simulink model "db3_7_Level_double"  (R2021a)
settings: Solver=VariableStepAuto  StartTime=0.0  StopTime=8  RelTol=1e-3
undefined symbols (not defined in the file): lambda2
libraries: dspsigops x15, dspquant2 x1
(part 2 of 4)

== system db3_7_Level_double/1st_Level_Decomp/HiD_Odd ==
  In_HiD_o : Inport  OutDataTypeStr=double  SampleTime=1/44100
  Add : Sum  AccumDataTypeStr=double  OutDataTypeStr=double
  Add1 : Sum  AccumDataTypeStr=double  OutDataTypeStr=double
  Delay{,1..3} (4 alike) : Delay  DelayLength=1  SampleTime=1/44100
  HiD_1 : Constant  Value=0.806891509  OutDataTypeStr=double  SampleTime=1/44100
  HiD_3 : Constant  Value=-0.13501102  OutDataTypeStr=double  SampleTime=1/44100
  HiD_5 : Constant  Value=0.035226292  OutDataTypeStr=double  SampleTime=1/44100
  Multiply : Product  OutDataTypeStr=double
  Multiply1 : Product  OutDataTypeStr=double
  Multiply2 : Product  OutDataTypeStr=double
  Rate Transition : RateTransition  OutPortSampleTime=1/44100
  Rate Transition1 : RateTransition  OutPortSampleTime=1/44100
  Out_HiD_o : Outport  OutDataTypeStr=double  SampleTime=1/44100  VectorParamsAs1DForOutWhenUnconnected=off
  wires:
  HiD_5/1 -> Multiply2/1
  HiD_3/1 -> Multiply1/1
  Add/1 -> Out_HiD_o/1
  Delay2/1 -> Add1/2
  Delay3/1 -> Add/2
  Add1/1 -> Delay3/1
  Multiply/1 -> Add/1
  HiD_1/1 -> Multiply/1
  Rate Transition/1 -> Delay1/1, Multiply1/2
  Multiply1/1 -> Add1/1
  Multiply2/1 -> Delay2/1
  Rate Transition1/1 -> Multiply2/2
  In_HiD_o/1 -> Multiply/2, Delay/1
  Delay/1 -> Rate Transition/1
  Delay1/1 -> Rate Transition1/1

== system db3_7_Level_double/1st_Level_Decomp/LoD_Even ==
  In_LoD_e : Inport  OutDataTypeStr=double  SampleTime=1/44100
  Add : Sum  AccumDataTypeStr=double  OutDataTypeStr=double
  Add1 : Sum  AccumDataTypeStr=double  OutDataTypeStr=double
  Delay{,1..3} (4 alike) : Delay  DelayLength=1  SampleTime=1/44100
  LoD_0 : Constant  Value=0.035226292  OutDataTypeStr=double  SampleTime=1/44100
  LoD_2 : Constant  Value=-0.13501102  OutDataTypeStr=double  SampleTime=1/44100
  LoD_4 : Constant  Value=0.806891509  OutDataTypeStr=double  SampleTime=1/44100
  Multiply : Product  OutDataTypeStr=double
  Multiply1 : Product  OutDataTypeStr=double
  Multiply2 : Product  OutDataTypeStr=double
  Rate Transition : RateTransition  OutPortSampleTime=1/44100
  Rate Transition1 : RateTransition  OutPortSampleTime=1/44100
  Out_LoD_e : Outport  OutDataTypeStr=double  SampleTime=1/44100  VectorParamsAs1DForOutWhenUnconnected=off
  wires:
  LoD_4/1 -> Multiply2/1
  LoD_2/1 -> Multiply1/1
  Add/1 -> Out_LoD_e/1
  Delay2/1 -> Add1/2
  Delay3/1 -> Add/2
  Add1/1 -> Delay3/1
  Multiply/1 -> Add/1
  LoD_0/1 -> Multiply/1
  Rate Transition/1 -> Delay1/1, Multiply1/2
  Multiply1/1 -> Add1/1
  Multiply2/1 -> Delay2/1
  Rate Transition1/1 -> Multiply2/2
  In_LoD_e/1 -> Delay/1, Multiply/2
  Delay/1 -> Rate Transition/1
  Delay1/1 -> Rate Transition1/1

== system db3_7_Level_double/1st_Level_Decomp/LoD_Odd ==
  In_LoD_o : Inport  OutDataTypeStr=double  SampleTime=1/44100
  Add : Sum  AccumDataTypeStr=double  OutDataTypeStr=double
  Add1 : Sum  AccumDataTypeStr=double  OutDataTypeStr=double
  Delay{,1..3} (4 alike) : Delay  DelayLength=1  SampleTime=1/44100
  LoD_1 : Constant  Value=-0.085441274  OutDataTypeStr=double  SampleTime=1/44100
  LoD_3 : Constant  Value=0.459877502  OutDataTypeStr=double  SampleTime=1/44100
  LoD_5 : Constant  Value=0.332670553  OutDataTypeStr=double  SampleTime=1/44100
  Multiply : Product  OutDataTypeStr=double
  Multiply1 : Product  OutDataTypeStr=double
  Multiply2 : Product  OutDataTypeStr=double
  Rate Transition : RateTransition  OutPortSampleTime=1/44100
  Rate Transition1 : RateTransition  OutPortSampleTime=1/44100
  Out_LoD_o : Outport  OutDataTypeStr=double  SampleTime=1/44100  VectorParamsAs1DForOutWhenUnconnected=off
  wires:
  LoD_5/1 -> Multiply2/1
  LoD_3/1 -> Multiply1/1
  Add/1 -> Out_LoD_o/1
  Delay2/1 -> Add1/2
  Delay3/1 -> Add/2
  Add1/1 -> Delay3/1
  Multiply/1 -> Add/1
  LoD_1/1 -> Multiply/1
  Rate Transition/1 -> Delay1/1, Multiply1/2
  Multiply1/1 -> Add1/1
  Multiply2/1 -> Delay2/1
  Rate Transition1/1 -> Multiply2/2
  In_LoD_o/1 -> Delay/1, Multiply/2
  Delay/1 -> Rate Transition/1
  Delay1/1 -> Rate Transition1/1

== system db3_7_Level_double/1st_Level_Recon/HiR_Even ==
  In_HiR_e : Inport  OutDataTypeStr=double  SampleTime=1/44100
  Add : Sum  AccumDataTypeStr=double  OutDataTypeStr=double
  Add1 : Sum  AccumDataTypeStr=double  OutDataTypeStr=double
  Delay : Delay  DelayLength=1  SampleTime=1/44100
  Delay1 : Delay  DelayLength=1  SampleTime=1/44100
  Delay2 : Delay  DelayLength=1  SampleTime=0.000022675736
  Delay3 : Delay  DelayLength=1  SampleTime=0.000022675736
  HiR_0 : Constant  Value=0.035226292  OutDataTypeStr=double  SampleTime=1/44100
  HiR_2 : Constant  Value=-0.13501102  OutDataTypeStr=double  SampleTime=1/44100
  HiR_4 : Constant  Value=0.806891509  OutDataTypeStr=double  SampleTime=1/44100
  Multiply : Product  OutDataTypeStr=double
  Multiply1 : Product  OutDataTypeStr=double
  Multiply2 : Product  OutDataTypeStr=double
  Rate Transition : RateTransition  OutPortSampleTime=1/44100
  Rate Transition1 : RateTransition  OutPortSampleTime=1/44100
  Out_HiR_e : Outport  OutDataTypeStr=double  SampleTime=1/44100  VectorParamsAs1DForOutWhenUnconnected=off
  wires:
  Delay3/1 -> Add/2
  In_HiR_e/1 -> Delay/1, Multiply/2
  HiR_4/1 -> Multiply2/1
  Multiply/1 -> Add/1
  Add1/1 -> Delay3/1
  Multiply2/1 -> Delay2/1
  Multiply1/1 -> Add1/1
  Delay2/1 -> Add1/2
  Add/1 -> Out_HiR_e/1
  HiR_0/1 -> Multiply/1
  HiR_2/1 -> Multiply1/1
  Delay1/1 -> Rate Transition1/1
  Rate Transition/1 -> Delay1/1, Multiply1/2
  Rate Transition1/1 -> Multiply2/2
  Delay/1 -> Rate Transition/1

== system db3_7_Level_double/1st_Level_Recon/HiR_Odd ==
  In_HiR_o : Inport  OutDataTypeStr=double  SampleTime=1/44100
  Add : Sum  AccumDataTypeStr=double  OutDataTypeStr=double
  Add1 : Sum  AccumDataTypeStr=double  OutDataTypeStr=double
  Delay{,1..3} (4 alike) : Delay  DelayLength=1  SampleTime=1/44100
  HiR_1 : Constant  Value=0.085441274  OutDataTypeStr=double  SampleTime=1/44100
  HiR_3 : Constant  Value=-0.459877502  OutDataTypeStr=double  SampleTime=1/44100
  HiR_5 : Constant  Value=-0.332670553  OutDataTypeStr=double  SampleTime=1/44100  LockScale=on
  Multiply : Product  OutDataTypeStr=double
  Multiply1 : Product  OutDataTypeStr=double
  Multiply2 : Product  OutDataTypeStr=double
  Rate Transition : RateTransition  OutPortSampleTime=1/44100
  Rate Transition1 : RateTransition  OutPortSampleTime=1/44100
  Out_HiR_o : Outport  OutDataTypeStr=double  SampleTime=1/44100  VectorParamsAs1DForOutWhenUnconnected=off
  wires:
  Delay/1 -> Rate Transition/1
  Rate Transition1/1 -> Multiply2/2
  Delay2/1 -> Add1/2
  HiR_1/1 -> Multiply/1
  Add/1 -> Out_HiR_o/1
  Delay1/1 -> Rate Transition1/1
  HiR_3/1 -> Multiply1/1
  Multiply1/1 -> Add1/1
  Rate Transition/1 -> Delay1/1, Multiply1/2
  Add1/1 -> Delay3/1
  Multiply/1 -> Add/1
  In_HiR_o/1 -> Delay/1, Multiply/2
  Multiply2/1 -> Delay2/1
  HiR_5/1 -> Multiply2/1
  Delay3/1 -> Add/2

== system db3_7_Level_double/1st_Level_Recon/LoR_Even ==
  In_LoR_e : Inport  OutDataTypeStr=double  SampleTime=1/44100
  Add : Sum  AccumDataTypeStr=double  OutDataTypeStr=double
  Add1 : Sum  AccumDataTypeStr=double  OutDataTypeStr=double
  Delay{,1..3} (4 alike) : Delay  DelayLength=1  SampleTime=1/44100
  LoR_0 : Constant  Value=0.332670553  OutDataTypeStr=double  SampleTime=1/44100
  LoR_2 : Constant  Value=0.459877502  OutDataTypeStr=double  SampleTime=1/44100
  LoR_4 : Constant  Value=-0.085441274  OutDataTypeStr=double  SampleTime=1/44100
  Multiply : Product  OutDataTypeStr=double
  Multiply1 : Product  OutDataTypeStr=double
  Multiply2 : Product  OutDataTypeStr=double
  Rate Transition : RateTransition  OutPortSampleTime=1/44100
  Rate Transition1 : RateTransition  OutPortSampleTime=1/44100
  Out_LoR_e : Outport  OutDataTypeStr=double  SampleTime=1/44100  VectorParamsAs1DForOutWhenUnconnected=off
  wires:
  Delay/1 -> Rate Transition/1
  Rate Transition1/1 -> Multiply2/2
  Delay2/1 -> Add1/2
  LoR_0/1 -> Multiply/1
  Add/1 -> Out_LoR_e/1
  Delay1/1 -> Rate Transition1/1
  LoR_2/1 -> Multiply1/1
  Multiply1/1 -> Add1/1
  Rate Transition/1 -> Delay1/1, Multiply1/2
  Add1/1 -> Delay3/1
  Multiply/1 -> Add/1
  In_LoR_e/1 -> Delay/1, Multiply/2
  Multiply2/1 -> Delay2/1
  LoR_4/1 -> Multiply2/1
  Delay3/1 -> Add/2

== system db3_7_Level_double/1st_Level_Recon/LoR_Odd ==
  In_LoR_o : Inport  OutDataTypeStr=double  SampleTime=1/44100
  Add : Sum  AccumDataTypeStr=double  OutDataTypeStr=double
  Add1 : Sum  AccumDataTypeStr=double  OutDataTypeStr=double
  Delay{,1..3} (4 alike) : Delay  DelayLength=1  SampleTime=1/44100
  LoR_1 : Constant  Value=0.806891509  OutDataTypeStr=double  SampleTime=1/44100
  LoR_3 : Constant  Value=-0.13501102  OutDataTypeStr=double  SampleTime=1/44100
  LoR_5 : Constant  Value=0.035226292  OutDataTypeStr=double  SampleTime=1/44100
  Multiply : Product  OutDataTypeStr=double
  Multiply1 : Product  OutDataTypeStr=double
  Multiply2 : Product  OutDataTypeStr=double
  Rate Transition : RateTransition  OutPortSampleTime=1/44100
  Rate Transition1 : RateTransition  OutPortSampleTime=1/44100
  Out_LoR_o : Outport  OutDataTypeStr=double  SampleTime=1/44100  VectorParamsAs1DForOutWhenUnconnected=off
  wires:
  Delay/1 -> Rate Transition/1
  Rate Transition1/1 -> Multiply2/2
  Delay2/1 -> Add1/2
  LoR_1/1 -> Multiply/1
  Add/1 -> Out_LoR_o/1
  Delay1/1 -> Rate Transition1/1
  LoR_3/1 -> Multiply1/1
  Multiply1/1 -> Add1/1
  Rate Transition/1 -> Delay1/1, Multiply1/2
  Add1/1 -> Delay3/1
  Multiply/1 -> Add/1
  In_LoR_o/1 -> Delay/1, Multiply/2
  Multiply2/1 -> Delay2/1
  LoR_5/1 -> Multiply2/1
  Delay3/1 -> Add/2

== system db3_7_Level_double/2nd_Level_Decomp/HiD_Even ==
  In_HiD_e : Inport  OutDataTypeStr=double  SampleTime=1/44100
  Add : Sum  AccumDataTypeStr=double  OutDataTypeStr=double
  Add1 : Sum  AccumDataTypeStr=double  OutDataTypeStr=double
  Delay{,1..3} (4 alike) : Delay  DelayLength=1  SampleTime=1/44100
  HiD_0 : Constant  Value=-0.332670553  OutDataTypeStr=double  SampleTime=1/44100
  HiD_2 : Constant  Value=-0.459877502  OutDataTypeStr=double  SampleTime=1/44100
  HiD_4 : Constant  Value=0.085441274  OutDataTypeStr=double  SampleTime=1/44100
  Multiply : Product  OutDataTypeStr=double
  Multiply1 : Product  OutDataTypeStr=double
  Multiply2 : Product  OutDataTypeStr=double
  Rate Transition : RateTransition  OutPortSampleTime=1/44100
  Rate Transition1 : RateTransition  OutPortSampleTime=1/44100
  Out_HiD_e : Outport  OutDataTypeStr=double  SampleTime=1/44100  VectorParamsAs1DForOutWhenUnconnected=off
  wires:
  In_HiD_e/1 -> Delay/1, Multiply/2
  Rate Transition/1 -> Delay1/1, Multiply1/2
  HiD_0/1 -> Multiply/1
  HiD_2/1 -> Multiply1/1
  Add/1 -> Out_HiD_e/1
  Rate Transition1/1 -> Multiply2/2
  HiD_4/1 -> Multiply2/1
  Multiply1/1 -> Add1/1
  Multiply2/1 -> Delay2/1
  Delay2/1 -> Add1/2
  Add1/1 -> Delay3/1
  Delay3/1 -> Add/2
  Multiply/1 -> Add/1
  Delay/1 -> Rate Transition/1
  Delay1/1 -> Rate Transition1/1

== system db3_7_Level_double/2nd_Level_Decomp/HiD_Odd ==
  In_HiD_o : Inport  OutDataTypeStr=double  SampleTime=1/44100
  Add : Sum  AccumDataTypeStr=double  OutDataTypeStr=double
  Add1 : Sum  AccumDataTypeStr=double  OutDataTypeStr=double
  Delay{,1..3} (4 alike) : Delay  DelayLength=1  SampleTime=1/44100
  HiD_1 : Constant  Value=0.806891509  OutDataTypeStr=double  SampleTime=1/44100
  HiD_3 : Constant  Value=-0.13501102  OutDataTypeStr=double  SampleTime=1/44100
  HiD_5 : Constant  Value=0.035226292  OutDataTypeStr=double  SampleTime=1/44100
  Multiply : Product  OutDataTypeStr=double
  Multiply1 : Product  OutDataTypeStr=double
  Multiply2 : Product  OutDataTypeStr=double
  Rate Transition : RateTransition  OutPortSampleTime=1/44100
  Rate Transition1 : RateTransition  OutPortSampleTime=1/44100
  Out_HiD_o : Outport  OutDataTypeStr=double  SampleTime=1/44100  VectorParamsAs1DForOutWhenUnconnected=off
  wires:
  HiD_5/1 -> Multiply2/1
  HiD_3/1 -> Multiply1/1
  Add/1 -> Out_HiD_o/1
  Delay2/1 -> Add1/2
  Delay3/1 -> Add/2
  Add1/1 -> Delay3/1
  Multiply/1 -> Add/1
  HiD_1/1 -> Multiply/1
  Rate Transition/1 -> Delay1/1, Multiply1/2
  Multiply1/1 -> Add1/1
  Multiply2/1 -> Delay2/1
  Rate Transition1/1 -> Multiply2/2
  In_HiD_o/1 -> Multiply/2, Delay/1
  Delay/1 -> Rate Transition/1
  Delay1/1 -> Rate Transition1/1

== system db3_7_Level_double/2nd_Level_Decomp/LoD_Even ==
  In_LoD_e : Inport  OutDataTypeStr=double  SampleTime=1/44100
  Add : Sum  AccumDataTypeStr=double  OutDataTypeStr=double
  Add1 : Sum  AccumDataTypeStr=double  OutDataTypeStr=double
  Delay{,1..3} (4 alike) : Delay  DelayLength=1  SampleTime=1/44100
  LoD_0 : Constant  Value=0.035226292  OutDataTypeStr=double  SampleTime=1/44100
  LoD_2 : Constant  Value=-0.13501102  OutDataTypeStr=double  SampleTime=1/44100
  LoD_4 : Constant  Value=0.806891509  OutDataTypeStr=double  SampleTime=1/44100
  Multiply : Product  OutDataTypeStr=double
  Multiply1 : Product  OutDataTypeStr=double
  Multiply2 : Product  OutDataTypeStr=double
  Rate Transition : RateTransition  OutPortSampleTime=1/44100
  Rate Transition1 : RateTransition  OutPortSampleTime=1/44100
  Out_LoD_e : Outport  OutDataTypeStr=double  SampleTime=1/44100  VectorParamsAs1DForOutWhenUnconnected=off
  wires:
  LoD_4/1 -> Multiply2/1
  LoD_2/1 -> Multiply1/1
  Add/1 -> Out_LoD_e/1
  Delay2/1 -> Add1/2
  Delay3/1 -> Add/2
  Add1/1 -> Delay3/1
  Multiply/1 -> Add/1
  LoD_0/1 -> Multiply/1
  Rate Transition/1 -> Delay1/1, Multiply1/2
  Multiply1/1 -> Add1/1
  Multiply2/1 -> Delay2/1
  Rate Transition1/1 -> Multiply2/2
  In_LoD_e/1 -> Delay/1, Multiply/2
  Delay/1 -> Rate Transition/1
  Delay1/1 -> Rate Transition1/1

== system db3_7_Level_double/2nd_Level_Decomp/LoD_Odd ==
  In_LoD_o : Inport  OutDataTypeStr=double  SampleTime=1/44100
  Add : Sum  AccumDataTypeStr=double  OutDataTypeStr=double
  Add1 : Sum  AccumDataTypeStr=double  OutDataTypeStr=double
  Delay{,1..3} (4 alike) : Delay  DelayLength=1  SampleTime=1/44100
  LoD_1 : Constant  Value=-0.085441274  OutDataTypeStr=double  SampleTime=1/44100
  LoD_3 : Constant  Value=0.459877502  OutDataTypeStr=double  SampleTime=1/44100
  LoD_5 : Constant  Value=0.332670553  OutDataTypeStr=double  SampleTime=1/44100
  Multiply : Product  OutDataTypeStr=double
  Multiply1 : Product  OutDataTypeStr=double
  Multiply2 : Product  OutDataTypeStr=double
  Rate Transition : RateTransition  OutPortSampleTime=1/44100
  Rate Transition1 : RateTransition  OutPortSampleTime=1/44100
  Out_LoD_o : Outport  OutDataTypeStr=double  SampleTime=1/44100  VectorParamsAs1DForOutWhenUnconnected=off
  wires:
  LoD_5/1 -> Multiply2/1
  LoD_3/1 -> Multiply1/1
  Add/1 -> Out_LoD_o/1
  Delay2/1 -> Add1/2
  Delay3/1 -> Add/2
  Add1/1 -> Delay3/1
  Multiply/1 -> Add/1
  LoD_1/1 -> Multiply/1
  Rate Transition/1 -> Delay1/1, Multiply1/2
  Multiply1/1 -> Add1/1
  Multiply2/1 -> Delay2/1
  Rate Transition1/1 -> Multiply2/2
  In_LoD_o/1 -> Delay/1, Multiply/2
  Delay/1 -> Rate Transition/1
  Delay1/1 -> Rate Transition1/1

== system db3_7_Level_double/2nd_Level_Recon/HiR_Even ==
  In_HiR_e : Inport  OutDataTypeStr=double  SampleTime=1/44100
  Add : Sum  AccumDataTypeStr=double  OutDataTypeStr=double
  Add1 : Sum  AccumDataTypeStr=double  OutDataTypeStr=double
  Delay : Delay  DelayLength=1  SampleTime=1/44100
  Delay1 : Delay  DelayLength=1  SampleTime=1/44100
  Delay2 : Delay  DelayLength=1  SampleTime=0.000022675736
  Delay3 : Delay  DelayLength=1  SampleTime=0.000022675736
  HiR_0 : Constant  Value=0.035226292  OutDataTypeStr=double  SampleTime=1/44100
  HiR_2 : Constant  Value=-0.13501102  OutDataTypeStr=double  SampleTime=1/44100
  HiR_4 : Constant  Value=0.806891509  OutDataTypeStr=double  SampleTime=1/44100
  Multiply : Product  OutDataTypeStr=double
  Multiply1 : Product  OutDataTypeStr=double
  Multiply2 : Product  OutDataTypeStr=double
  Rate Transition : RateTransition  OutPortSampleTime=1/44100
  Rate Transition1 : RateTransition  OutPortSampleTime=1/44100
  Out_HiR_e : Outport  OutDataTypeStr=double  SampleTime=1/44100  VectorParamsAs1DForOutWhenUnconnected=off
  wires:
  Delay3/1 -> Add/2
  In_HiR_e/1 -> Delay/1, Multiply/2
  HiR_4/1 -> Multiply2/1
  Multiply/1 -> Add/1
  Add1/1 -> Delay3/1
  Multiply2/1 -> Delay2/1
  Multiply1/1 -> Add1/1
  Delay2/1 -> Add1/2
  Add/1 -> Out_HiR_e/1
  HiR_0/1 -> Multiply/1
  HiR_2/1 -> Multiply1/1
  Delay1/1 -> Rate Transition1/1
  Rate Transition/1 -> Delay1/1, Multiply1/2
  Rate Transition1/1 -> Multiply2/2
  Delay/1 -> Rate Transition/1

== system db3_7_Level_double/2nd_Level_Recon/HiR_Odd ==
  In_HiR_o : Inport  OutDataTypeStr=double  SampleTime=1/44100
  Add : Sum  AccumDataTypeStr=double  OutDataTypeStr=double
  Add1 : Sum  AccumDataTypeStr=double  OutDataTypeStr=double
  Delay{,1..3} (4 alike) : Delay  DelayLength=1  SampleTime=1/44100
  HiR_1 : Constant  Value=0.085441274  OutDataTypeStr=double  SampleTime=1/44100
  HiR_3 : Constant  Value=-0.459877502  OutDataTypeStr=double  SampleTime=1/44100
  HiR_5 : Constant  Value=-0.332670553  OutDataTypeStr=double  SampleTime=1/44100  LockScale=on
  Multiply : Product  OutDataTypeStr=double
  Multiply1 : Product  OutDataTypeStr=double
  Multiply2 : Product  OutDataTypeStr=double
  Rate Transition : RateTransition  OutPortSampleTime=1/44100
  Rate Transition1 : RateTransition  OutPortSampleTime=1/44100
  Out_HiR_o : Outport  OutDataTypeStr=double  SampleTime=1/44100  VectorParamsAs1DForOutWhenUnconnected=off
  wires:
  Delay/1 -> Rate Transition/1
  Rate Transition1/1 -> Multiply2/2
  Delay2/1 -> Add1/2
  HiR_1/1 -> Multiply/1
  Add/1 -> Out_HiR_o/1
  Delay1/1 -> Rate Transition1/1
  HiR_3/1 -> Multiply1/1
  Multiply1/1 -> Add1/1
  Rate Transition/1 -> Delay1/1, Multiply1/2
  Add1/1 -> Delay3/1
  Multiply/1 -> Add/1
  In_HiR_o/1 -> Delay/1, Multiply/2
  Multiply2/1 -> Delay2/1
  HiR_5/1 -> Multiply2/1
  Delay3/1 -> Add/2

== system db3_7_Level_double/2nd_Level_Recon/LoR_Even ==
  In_LoR_e : Inport  OutDataTypeStr=double  SampleTime=1/44100
  Add : Sum  AccumDataTypeStr=double  OutDataTypeStr=double
  Add1 : Sum  AccumDataTypeStr=double  OutDataTypeStr=double
  Delay{,1..3} (4 alike) : Delay  DelayLength=1  SampleTime=1/44100
  LoR_0 : Constant  Value=0.332670553  OutDataTypeStr=double  SampleTime=1/44100
  LoR_2 : Constant  Value=0.459877502  OutDataTypeStr=double  SampleTime=1/44100
  LoR_4 : Constant  Value=-0.085441274  OutDataTypeStr=double  SampleTime=1/44100
  Multiply : Product  OutDataTypeStr=double
  Multiply1 : Product  OutDataTypeStr=double
  Multiply2 : Product  OutDataTypeStr=double
  Rate Transition : RateTransition  OutPortSampleTime=1/44100
  Rate Transition1 : RateTransition  OutPortSampleTime=1/44100
  Out_LoR_e : Outport  OutDataTypeStr=double  SampleTime=1/44100  VectorParamsAs1DForOutWhenUnconnected=off
  wires:
  Delay/1 -> Rate Transition/1
  Rate Transition1/1 -> Multiply2/2
  Delay2/1 -> Add1/2
  LoR_0/1 -> Multiply/1
  Add/1 -> Out_LoR_e/1
  Delay1/1 -> Rate Transition1/1
  LoR_2/1 -> Multiply1/1
  Multiply1/1 -> Add1/1
  Rate Transition/1 -> Delay1/1, Multiply1/2
  Add1/1 -> Delay3/1
  Multiply/1 -> Add/1
  In_LoR_e/1 -> Delay/1, Multiply/2
  Multiply2/1 -> Delay2/1
  LoR_4/1 -> Multiply2/1
  Delay3/1 -> Add/2

== system db3_7_Level_double/2nd_Level_Recon/LoR_Odd ==
  In_LoR_o : Inport  OutDataTypeStr=double  SampleTime=1/44100
  Add : Sum  AccumDataTypeStr=double  OutDataTypeStr=double
  Add1 : Sum  AccumDataTypeStr=double  OutDataTypeStr=double
  Delay{,1..3} (4 alike) : Delay  DelayLength=1  SampleTime=1/44100
  LoR_1 : Constant  Value=0.806891509  OutDataTypeStr=double  SampleTime=1/44100
  LoR_3 : Constant  Value=-0.13501102  OutDataTypeStr=double  SampleTime=1/44100
  LoR_5 : Constant  Value=0.035226292  OutDataTypeStr=double  SampleTime=1/44100
  Multiply : Product  OutDataTypeStr=double
  Multiply1 : Product  OutDataTypeStr=double
  Multiply2 : Product  OutDataTypeStr=double
  Rate Transition : RateTransition  OutPortSampleTime=1/44100
  Rate Transition1 : RateTransition  OutPortSampleTime=1/44100
  Out_LoR_o : Outport  OutDataTypeStr=double  SampleTime=1/44100  VectorParamsAs1DForOutWhenUnconnected=off
  wires:
  Delay/1 -> Rate Transition/1
  Rate Transition1/1 -> Multiply2/2
  Delay2/1 -> Add1/2
  LoR_1/1 -> Multiply/1
  Add/1 -> Out_LoR_o/1
  Delay1/1 -> Rate Transition1/1
  LoR_3/1 -> Multiply1/1
  Multiply1/1 -> Add1/1
  Rate Transition/1 -> Delay1/1, Multiply1/2
  Add1/1 -> Delay3/1
  Multiply/1 -> Add/1
  In_LoR_o/1 -> Delay/1, Multiply/2
  Multiply2/1 -> Delay2/1
  LoR_5/1 -> Multiply2/1
  Delay3/1 -> Add/2

== system db3_7_Level_double/3rd_Level_Decomp/HiD_Even ==
  In_HiD_e : Inport  OutDataTypeStr=double  SampleTime=1/44100
  Add : Sum  AccumDataTypeStr=double  OutDataTypeStr=double
  Add1 : Sum  AccumDataTypeStr=double  OutDataTypeStr=double
  Delay{,1..3} (4 alike) : Delay  DelayLength=1  SampleTime=1/44100
  HiD_0 : Constant  Value=-0.332670553  OutDataTypeStr=double  SampleTime=1/44100
  HiD_2 : Constant  Value=-0.459877502  OutDataTypeStr=double  SampleTime=1/44100
  HiD_4 : Constant  Value=0.085441274  OutDataTypeStr=double  SampleTime=1/44100
  Multiply : Product  OutDataTypeStr=double
  Multiply1 : Product  OutDataTypeStr=double
  Multiply2 : Product  OutDataTypeStr=double
  Rate Transition : RateTransition  OutPortSampleTime=1/44100
  Rate Transition1 : RateTransition  OutPortSampleTime=1/44100
  Out_HiD_e : Outport  OutDataTypeStr=double  SampleTime=1/44100  VectorParamsAs1DForOutWhenUnconnected=off
  wires:
  In_HiD_e/1 -> Delay/1, Multiply/2
  Rate Transition/1 -> Delay1/1, Multiply1/2
  HiD_0/1 -> Multiply/1
  HiD_2/1 -> Multiply1/1
  Add/1 -> Out_HiD_e/1
  Rate Transition1/1 -> Multiply2/2
  HiD_4/1 -> Multiply2/1
  Multiply1/1 -> Add1/1
  Multiply2/1 -> Delay2/1
  Delay2/1 -> Add1/2
  Add1/1 -> Delay3/1
  Delay3/1 -> Add/2
  Multiply/1 -> Add/1
  Delay/1 -> Rate Transition/1
  Delay1/1 -> Rate Transition1/1

== system db3_7_Level_double/3rd_Level_Decomp/HiD_Odd ==
  In_HiD_o : Inport  OutDataTypeStr=double  SampleTime=1/44100
  Add : Sum  AccumDataTypeStr=double  OutDataTypeStr=double
  Add1 : Sum  AccumDataTypeStr=double  OutDataTypeStr=double
  Delay{,1..3} (4 alike) : Delay  DelayLength=1  SampleTime=1/44100
  HiD_1 : Constant  Value=0.806891509  OutDataTypeStr=double  SampleTime=1/44100
  HiD_3 : Constant  Value=-0.13501102  OutDataTypeStr=double  SampleTime=1/44100
  HiD_5 : Constant  Value=0.035226292  OutDataTypeStr=double  SampleTime=1/44100
  Multiply : Product  OutDataTypeStr=double
  Multiply1 : Product  OutDataTypeStr=double
  Multiply2 : Product  OutDataTypeStr=double
  Rate Transition : RateTransition  OutPortSampleTime=1/44100
  Rate Transition1 : RateTransition  OutPortSampleTime=1/44100
  Out_HiD_o : Outport  OutDataTypeStr=double  SampleTime=1/44100  VectorParamsAs1DForOutWhenUnconnected=off
  wires:
  HiD_5/1 -> Multiply2/1
  HiD_3/1 -> Multiply1/1
  Add/1 -> Out_HiD_o/1
  Delay2/1 -> Add1/2
  Delay3/1 -> Add/2
  Add1/1 -> Delay3/1
  Multiply/1 -> Add/1
  HiD_1/1 -> Multiply/1
  Rate Transition/1 -> Delay1/1, Multiply1/2
  Multiply1/1 -> Add1/1
  Multiply2/1 -> Delay2/1
  Rate Transition1/1 -> Multiply2/2
  In_HiD_o/1 -> Multiply/2, Delay/1
  Delay/1 -> Rate Transition/1
  Delay1/1 -> Rate Transition1/1

== system db3_7_Level_double/3rd_Level_Decomp/LoD_Even ==
  In_LoD_e : Inport  OutDataTypeStr=double  SampleTime=1/44100
  Add : Sum  AccumDataTypeStr=double  OutDataTypeStr=double
  Add1 : Sum  AccumDataTypeStr=double  OutDataTypeStr=double
  Delay{,1..3} (4 alike) : Delay  DelayLength=1  SampleTime=1/44100
  LoD_0 : Constant  Value=0.035226292  OutDataTypeStr=double  SampleTime=1/44100
  LoD_2 : Constant  Value=-0.13501102  OutDataTypeStr=double  SampleTime=1/44100
  LoD_4 : Constant  Value=0.806891509  OutDataTypeStr=double  SampleTime=1/44100
  Multiply : Product  OutDataTypeStr=double
  Multiply1 : Product  OutDataTypeStr=double
  Multiply2 : Product  OutDataTypeStr=double
  Rate Transition : RateTransition  OutPortSampleTime=1/44100
  Rate Transition1 : RateTransition  OutPortSampleTime=1/44100
  Out_LoD_e : Outport  OutDataTypeStr=double  SampleTime=1/44100  VectorParamsAs1DForOutWhenUnconnected=off
  wires:
  LoD_4/1 -> Multiply2/1
  LoD_2/1 -> Multiply1/1
  Add/1 -> Out_LoD_e/1
  Delay2/1 -> Add1/2
  Delay3/1 -> Add/2
  Add1/1 -> Delay3/1
  Multiply/1 -> Add/1
  LoD_0/1 -> Multiply/1
  Rate Transition/1 -> Delay1/1, Multiply1/2
  Multiply1/1 -> Add1/1
  Multiply2/1 -> Delay2/1
  Rate Transition1/1 -> Multiply2/2
  In_LoD_e/1 -> Delay/1, Multiply/2
  Delay/1 -> Rate Transition/1
  Delay1/1 -> Rate Transition1/1

== system db3_7_Level_double/3rd_Level_Decomp/LoD_Odd ==
  In_LoD_o : Inport  OutDataTypeStr=double  SampleTime=1/44100
  Add : Sum  AccumDataTypeStr=double  OutDataTypeStr=double
  Add1 : Sum  AccumDataTypeStr=double  OutDataTypeStr=double
  Delay{,1..3} (4 alike) : Delay  DelayLength=1  SampleTime=1/44100
  LoD_1 : Constant  Value=-0.085441274  OutDataTypeStr=double  SampleTime=1/44100
  LoD_3 : Constant  Value=0.459877502  OutDataTypeStr=double  SampleTime=1/44100
  LoD_5 : Constant  Value=0.332670553  OutDataTypeStr=double  SampleTime=1/44100
  Multiply : Product  OutDataTypeStr=double
  Multiply1 : Product  OutDataTypeStr=double
  Multiply2 : Product  OutDataTypeStr=double
  Rate Transition : RateTransition  OutPortSampleTime=1/44100
  Rate Transition1 : RateTransition  OutPortSampleTime=1/44100
  Out_LoD_o : Outport  OutDataTypeStr=double  SampleTime=1/44100  VectorParamsAs1DForOutWhenUnconnected=off
  wires:
  LoD_5/1 -> Multiply2/1
  LoD_3/1 -> Multiply1/1
  Add/1 -> Out_LoD_o/1
  Delay2/1 -> Add1/2
  Delay3/1 -> Add/2
  Add1/1 -> Delay3/1
  Multiply/1 -> Add/1
  LoD_1/1 -> Multiply/1
  Rate Transition/1 -> Delay1/1, Multiply1/2
  Multiply1/1 -> Add1/1
  Multiply2/1 -> Delay2/1
  Rate Transition1/1 -> Multiply2/2
  In_LoD_o/1 -> Delay/1, Multiply/2
  Delay/1 -> Rate Transition/1
  Delay1/1 -> Rate Transition1/1

== system db3_7_Level_double/3rd_Level_Recon/HiR_Even ==
  In_HiR_e : Inport  OutDataTypeStr=double  SampleTime=1/44100
  Add : Sum  AccumDataTypeStr=double  OutDataTypeStr=double
  Add1 : Sum  AccumDataTypeStr=double  OutDataTypeStr=double
  Delay : Delay  DelayLength=1  SampleTime=1/44100
  Delay1 : Delay  DelayLength=1  SampleTime=1/44100
  Delay2 : Delay  DelayLength=1  SampleTime=0.000022675736
  Delay3 : Delay  DelayLength=1  SampleTime=0.000022675736
  HiR_0 : Constant  Value=0.035226292  OutDataTypeStr=double  SampleTime=1/44100
  HiR_2 : Constant  Value=-0.13501102  OutDataTypeStr=double  SampleTime=1/44100
  HiR_4 : Constant  Value=0.806891509  OutDataTypeStr=double  SampleTime=1/44100
  Multiply : Product  OutDataTypeStr=double
  Multiply1 : Product  OutDataTypeStr=double
  Multiply2 : Product  OutDataTypeStr=double
  Rate Transition : RateTransition  OutPortSampleTime=1/44100
  Rate Transition1 : RateTransition  OutPortSampleTime=1/44100
  Out_HiR_e : Outport  OutDataTypeStr=double  SampleTime=1/44100  VectorParamsAs1DForOutWhenUnconnected=off
  wires:
  Delay3/1 -> Add/2
  In_HiR_e/1 -> Delay/1, Multiply/2
  HiR_4/1 -> Multiply2/1
  Multiply/1 -> Add/1
  Add1/1 -> Delay3/1
  Multiply2/1 -> Delay2/1
  Multiply1/1 -> Add1/1
  Delay2/1 -> Add1/2
  Add/1 -> Out_HiR_e/1
  HiR_0/1 -> Multiply/1
  HiR_2/1 -> Multiply1/1
  Delay1/1 -> Rate Transition1/1
  Rate Transition/1 -> Delay1/1, Multiply1/2
  Rate Transition1/1 -> Multiply2/2
  Delay/1 -> Rate Transition/1

== system db3_7_Level_double/3rd_Level_Recon/HiR_Odd ==
  In_HiR_o : Inport  OutDataTypeStr=double  SampleTime=1/44100
  Add : Sum  AccumDataTypeStr=double  OutDataTypeStr=double
  Add1 : Sum  AccumDataTypeStr=double  OutDataTypeStr=double
  Delay{,1..3} (4 alike) : Delay  DelayLength=1  SampleTime=1/44100
  HiR_1 : Constant  Value=0.085441274  OutDataTypeStr=double  SampleTime=1/44100
  HiR_3 : Constant  Value=-0.459877502  OutDataTypeStr=double  SampleTime=1/44100
  HiR_5 : Constant  Value=-0.332670553  OutDataTypeStr=double  SampleTime=1/44100  LockScale=on
  Multiply : Product  OutDataTypeStr=double
  Multiply1 : Product  OutDataTypeStr=double
  Multiply2 : Product  OutDataTypeStr=double
  Rate Transition : RateTransition  OutPortSampleTime=1/44100
  Rate Transition1 : RateTransition  OutPortSampleTime=1/44100
  Out_HiR_o : Outport  OutDataTypeStr=double  SampleTime=1/44100  VectorParamsAs1DForOutWhenUnconnected=off
  wires:
  Delay/1 -> Rate Transition/1
  Rate Transition1/1 -> Multiply2/2
  Delay2/1 -> Add1/2
  HiR_1/1 -> Multiply/1
  Add/1 -> Out_HiR_o/1
  Delay1/1 -> Rate Transition1/1
  HiR_3/1 -> Multiply1/1
  Multiply1/1 -> Add1/1
  Rate Transition/1 -> Delay1/1, Multiply1/2
  Add1/1 -> Delay3/1
  Multiply/1 -> Add/1
  In_HiR_o/1 -> Delay/1, Multiply/2
  Multiply2/1 -> Delay2/1
  HiR_5/1 -> Multiply2/1
  Delay3/1 -> Add/2

== system db3_7_Level_double/3rd_Level_Recon/LoR_Even ==
  In_LoR_e : Inport  OutDataTypeStr=double  SampleTime=1/44100
  Add : Sum  AccumDataTypeStr=double  OutDataTypeStr=double
  Add1 : Sum  AccumDataTypeStr=double  OutDataTypeStr=double
  Delay{,1..3} (4 alike) : Delay  DelayLength=1  SampleTime=1/44100
  LoR_0 : Constant  Value=0.332670553  OutDataTypeStr=double  SampleTime=1/44100
  LoR_2 : Constant  Value=0.459877502  OutDataTypeStr=double  SampleTime=1/44100
  LoR_4 : Constant  Value=-0.085441274  OutDataTypeStr=double  SampleTime=1/44100
  Multiply : Product  OutDataTypeStr=double
  Multiply1 : Product  OutDataTypeStr=double
  Multiply2 : Product  OutDataTypeStr=double
  Rate Transition : RateTransition  OutPortSampleTime=1/44100
  Rate Transition1 : RateTransition  OutPortSampleTime=1/44100
  Out_LoR_e : Outport  OutDataTypeStr=double  SampleTime=1/44100  VectorParamsAs1DForOutWhenUnconnected=off
  wires:
  Delay/1 -> Rate Transition/1
  Rate Transition1/1 -> Multiply2/2
  Delay2/1 -> Add1/2
  LoR_0/1 -> Multiply/1
  Add/1 -> Out_LoR_e/1
  Delay1/1 -> Rate Transition1/1
  LoR_2/1 -> Multiply1/1
  Multiply1/1 -> Add1/1
  Rate Transition/1 -> Delay1/1, Multiply1/2
  Add1/1 -> Delay3/1
  Multiply/1 -> Add/1
  In_LoR_e/1 -> Delay/1, Multiply/2
  Multiply2/1 -> Delay2/1
  LoR_4/1 -> Multiply2/1
  Delay3/1 -> Add/2

== system db3_7_Level_double/3rd_Level_Recon/LoR_Odd ==
  In_LoR_o : Inport  OutDataTypeStr=double  SampleTime=1/44100
  Add : Sum  AccumDataTypeStr=double  OutDataTypeStr=double
  Add1 : Sum  AccumDataTypeStr=double  OutDataTypeStr=double
  Delay{,1..3} (4 alike) : Delay  DelayLength=1  SampleTime=1/44100
  LoR_1 : Constant  Value=0.806891509  OutDataTypeStr=double  SampleTime=1/44100
  LoR_3 : Constant  Value=-0.13501102  OutDataTypeStr=double  SampleTime=1/44100
  LoR_5 : Constant  Value=0.035226292  OutDataTypeStr=double  SampleTime=1/44100
  Multiply : Product  OutDataTypeStr=double
  Multiply1 : Product  OutDataTypeStr=double
  Multiply2 : Product  OutDataTypeStr=double
  Rate Transition : RateTransition  OutPortSampleTime=1/44100
  Rate Transition1 : RateTransition  OutPortSampleTime=1/44100
  Out_LoR_o : Outport  OutDataTypeStr=double  SampleTime=1/44100  VectorParamsAs1DForOutWhenUnconnected=off
  wires:
  Delay/1 -> Rate Transition/1
  Rate Transition1/1 -> Multiply2/2
  Delay2/1 -> Add1/2
  LoR_1/1 -> Multiply/1
  Add/1 -> Out_LoR_o/1
  Delay1/1 -> Rate Transition1/1
  LoR_3/1 -> Multiply1/1
  Multiply1/1 -> Add1/1
  Rate Transition/1 -> Delay1/1, Multiply1/2
  Add1/1 -> Delay3/1
  Multiply/1 -> Add/1
  In_LoR_o/1 -> Delay/1, Multiply/2
  Multiply2/1 -> Delay2/1
  LoR_5/1 -> Multiply2/1
  Delay3/1 -> Add/2

== system db3_7_Level_double/4th_Level_Decomp/HiD_Even ==
  In_HiD_e : Inport  OutDataTypeStr=double  SampleTime=1/44100
  Add : Sum  AccumDataTypeStr=double  OutDataTypeStr=double
  Add1 : Sum  AccumDataTypeStr=double  OutDataTypeStr=double
  Delay{,1..3} (4 alike) : Delay  DelayLength=1  SampleTime=1/44100
  HiD_0 : Constant  Value=-0.332670553  OutDataTypeStr=double  SampleTime=1/44100
  HiD_2 : Constant  Value=-0.459877502  OutDataTypeStr=double  SampleTime=1/44100
  HiD_4 : Constant  Value=0.085441274  OutDataTypeStr=double  SampleTime=1/44100
  Multiply : Product  OutDataTypeStr=double
  Multiply1 : Product  OutDataTypeStr=double
  Multiply2 : Product  OutDataTypeStr=double
  Rate Transition : RateTransition  OutPortSampleTime=1/44100
  Rate Transition1 : RateTransition  OutPortSampleTime=1/44100
  Out_HiD_e : Outport  OutDataTypeStr=double  SampleTime=1/44100  VectorParamsAs1DForOutWhenUnconnected=off
  wires:
  In_HiD_e/1 -> Delay/1, Multiply/2
  Rate Transition/1 -> Delay1/1, Multiply1/2
  HiD_0/1 -> Multiply/1
  HiD_2/1 -> Multiply1/1
  Add/1 -> Out_HiD_e/1
  Rate Transition1/1 -> Multiply2/2
  HiD_4/1 -> Multiply2/1
  Multiply1/1 -> Add1/1
  Multiply2/1 -> Delay2/1
  Delay2/1 -> Add1/2
  Add1/1 -> Delay3/1
  Delay3/1 -> Add/2
  Multiply/1 -> Add/1
  Delay/1 -> Rate Transition/1
  Delay1/1 -> Rate Transition1/1

== system db3_7_Level_double/4th_Level_Decomp/HiD_Odd ==
  In_HiD_o : Inport  OutDataTypeStr=double  SampleTime=1/44100
  Add : Sum  AccumDataTypeStr=double  OutDataTypeStr=double
  Add1 : Sum  AccumDataTypeStr=double  OutDataTypeStr=double
  Delay{,1..3} (4 alike) : Delay  DelayLength=1  SampleTime=1/44100
  HiD_1 : Constant  Value=0.806891509  OutDataTypeStr=double  SampleTime=1/44100
  HiD_3 : Constant  Value=-0.13501102  OutDataTypeStr=double  SampleTime=1/44100
  HiD_5 : Constant  Value=0.035226292  OutDataTypeStr=double  SampleTime=1/44100
  Multiply : Product  OutDataTypeStr=double
  Multiply1 : Product  OutDataTypeStr=double
  Multiply2 : Product  OutDataTypeStr=double
  Rate Transition : RateTransition  OutPortSampleTime=1/44100
  Rate Transition1 : RateTransition  OutPortSampleTime=1/44100
  Out_HiD_o : Outport  OutDataTypeStr=double  SampleTime=1/44100  VectorParamsAs1DForOutWhenUnconnected=off
  wires:
  HiD_5/1 -> Multiply2/1
  HiD_3/1 -> Multiply1/1
  Add/1 -> Out_HiD_o/1
  Delay2/1 -> Add1/2
  Delay3/1 -> Add/2
  Add1/1 -> Delay3/1
  Multiply/1 -> Add/1
  HiD_1/1 -> Multiply/1
  Rate Transition/1 -> Delay1/1, Multiply1/2
  Multiply1/1 -> Add1/1
  Multiply2/1 -> Delay2/1
  Rate Transition1/1 -> Multiply2/2
  In_HiD_o/1 -> Multiply/2, Delay/1
  Delay/1 -> Rate Transition/1
  Delay1/1 -> Rate Transition1/1

== system db3_7_Level_double/4th_Level_Decomp/LoD_Even ==
  In_LoD_e : Inport  OutDataTypeStr=double  SampleTime=1/44100
  Add : Sum  AccumDataTypeStr=double  OutDataTypeStr=double
  Add1 : Sum  AccumDataTypeStr=double  OutDataTypeStr=double
  Delay{,1..3} (4 alike) : Delay  DelayLength=1  SampleTime=1/44100
  LoD_0 : Constant  Value=0.035226292  OutDataTypeStr=double  SampleTime=1/44100
  LoD_2 : Constant  Value=-0.13501102  OutDataTypeStr=double  SampleTime=1/44100
  LoD_4 : Constant  Value=0.806891509  OutDataTypeStr=double  SampleTime=1/44100
  Multiply : Product  OutDataTypeStr=double
  Multiply1 : Product  OutDataTypeStr=double
  Multiply2 : Product  OutDataTypeStr=double
  Rate Transition : RateTransition  OutPortSampleTime=1/44100
  Rate Transition1 : RateTransition  OutPortSampleTime=1/44100
  Out_LoD_e : Outport  OutDataTypeStr=double  SampleTime=1/44100  VectorParamsAs1DForOutWhenUnconnected=off
  wires:
  LoD_4/1 -> Multiply2/1
  LoD_2/1 -> Multiply1/1
  Add/1 -> Out_LoD_e/1
  Delay2/1 -> Add1/2
  Delay3/1 -> Add/2
  Add1/1 -> Delay3/1
  Multiply/1 -> Add/1
  LoD_0/1 -> Multiply/1
  Rate Transition/1 -> Delay1/1, Multiply1/2
  Multiply1/1 -> Add1/1
  Multiply2/1 -> Delay2/1
  Rate Transition1/1 -> Multiply2/2
  In_LoD_e/1 -> Delay/1, Multiply/2
  Delay/1 -> Rate Transition/1
  Delay1/1 -> Rate Transition1/1

== system db3_7_Level_double/4th_Level_Decomp/LoD_Odd ==
  In_LoD_o : Inport  OutDataTypeStr=double  SampleTime=1/44100
  Add : Sum  AccumDataTypeStr=double  OutDataTypeStr=double
  Add1 : Sum  AccumDataTypeStr=double  OutDataTypeStr=double
  Delay{,1..3} (4 alike) : Delay  DelayLength=1  SampleTime=1/44100
  LoD_1 : Constant  Value=-0.085441274  OutDataTypeStr=double  SampleTime=1/44100
  LoD_3 : Constant  Value=0.459877502  OutDataTypeStr=double  SampleTime=1/44100
  LoD_5 : Constant  Value=0.332670553  OutDataTypeStr=double  SampleTime=1/44100
  Multiply : Product  OutDataTypeStr=double
  Multiply1 : Product  OutDataTypeStr=double
  Multiply2 : Product  OutDataTypeStr=double
  Rate Transition : RateTransition  OutPortSampleTime=1/44100
  Rate Transition1 : RateTransition  OutPortSampleTime=1/44100
  Out_LoD_o : Outport  OutDataTypeStr=double  SampleTime=1/44100  VectorParamsAs1DForOutWhenUnconnected=off
  wires:
  LoD_5/1 -> Multiply2/1
  LoD_3/1 -> Multiply1/1
  Add/1 -> Out_LoD_o/1
  Delay2/1 -> Add1/2
  Delay3/1 -> Add/2
  Add1/1 -> Delay3/1
  Multiply/1 -> Add/1
  LoD_1/1 -> Multiply/1
  Rate Transition/1 -> Delay1/1, Multiply1/2
  Multiply1/1 -> Add1/1
  Multiply2/1 -> Delay2/1
  Rate Transition1/1 -> Multiply2/2
  In_LoD_o/1 -> Delay/1, Multiply/2
  Delay/1 -> Rate Transition/1
  Delay1/1 -> Rate Transition1/1

== system db3_7_Level_double/4th_Level_Recon/HiR_Even ==
  In_HiR_e : Inport  OutDataTypeStr=double  SampleTime=1/44100
  Add : Sum  AccumDataTypeStr=double  OutDataTypeStr=double
  Add1 : Sum  AccumDataTypeStr=double  OutDataTypeStr=double
  Delay : Delay  DelayLength=1  SampleTime=1/44100
  Delay1 : Delay  DelayLength=1  SampleTime=1/44100
  Delay2 : Delay  DelayLength=1  SampleTime=0.000022675736
  Delay3 : Delay  DelayLength=1  SampleTime=0.000022675736
  HiR_0 : Constant  Value=0.035226292  OutDataTypeStr=double  SampleTime=1/44100
  HiR_2 : Constant  Value=-0.13501102  OutDataTypeStr=double  SampleTime=1/44100
  HiR_4 : Constant  Value=0.806891509  OutDataTypeStr=double  SampleTime=1/44100
  Multiply : Product  OutDataTypeStr=double
  Multiply1 : Product  OutDataTypeStr=double
  Multiply2 : Product  OutDataTypeStr=double
  Rate Transition : RateTransition  OutPortSampleTime=1/44100
  Rate Transition1 : RateTransition  OutPortSampleTime=1/44100
  Out_HiR_e : Outport  OutDataTypeStr=double  SampleTime=1/44100  VectorParamsAs1DForOutWhenUnconnected=off
  wires:
  Delay3/1 -> Add/2
  In_HiR_e/1 -> Delay/1, Multiply/2
  HiR_4/1 -> Multiply2/1
  Multiply/1 -> Add/1
  Add1/1 -> Delay3/1
  Multiply2/1 -> Delay2/1
  Multiply1/1 -> Add1/1
  Delay2/1 -> Add1/2
  Add/1 -> Out_HiR_e/1
  HiR_0/1 -> Multiply/1
  HiR_2/1 -> Multiply1/1
  Delay1/1 -> Rate Transition1/1
  Rate Transition/1 -> Delay1/1, Multiply1/2
  Rate Transition1/1 -> Multiply2/2
  Delay/1 -> Rate Transition/1

== system db3_7_Level_double/4th_Level_Recon/HiR_Odd ==
  In_HiR_o : Inport  OutDataTypeStr=double  SampleTime=1/44100
  Add : Sum  AccumDataTypeStr=double  OutDataTypeStr=double
  Add1 : Sum  AccumDataTypeStr=double  OutDataTypeStr=double
  Delay{,1..3} (4 alike) : Delay  DelayLength=1  SampleTime=1/44100
  HiR_1 : Constant  Value=0.085441274  OutDataTypeStr=double  SampleTime=1/44100
  HiR_3 : Constant  Value=-0.459877502  OutDataTypeStr=double  SampleTime=1/44100
  HiR_5 : Constant  Value=-0.332670553  OutDataTypeStr=double  SampleTime=1/44100  LockScale=on
  Multiply : Product  OutDataTypeStr=double
  Multiply1 : Product  OutDataTypeStr=double
  Multiply2 : Product  OutDataTypeStr=double
  Rate Transition : RateTransition  OutPortSampleTime=1/44100
  Rate Transition1 : RateTransition  OutPortSampleTime=1/44100
  Out_HiR_o : Outport  OutDataTypeStr=double  SampleTime=1/44100  VectorParamsAs1DForOutWhenUnconnected=off
  wires:
  Delay/1 -> Rate Transition/1
  Rate Transition1/1 -> Multiply2/2
  Delay2/1 -> Add1/2
  HiR_1/1 -> Multiply/1
  Add/1 -> Out_HiR_o/1
  Delay1/1 -> Rate Transition1/1
  HiR_3/1 -> Multiply1/1
  Multiply1/1 -> Add1/1
  Rate Transition/1 -> Delay1/1, Multiply1/2
  Add1/1 -> Delay3/1
  Multiply/1 -> Add/1
  In_HiR_o/1 -> Delay/1, Multiply/2
  Multiply2/1 -> Delay2/1
  HiR_5/1 -> Multiply2/1
  Delay3/1 -> Add/2

== system db3_7_Level_double/4th_Level_Recon/LoR_Even ==
  In_LoR_e : Inport  OutDataTypeStr=double  SampleTime=1/44100
  Add : Sum  AccumDataTypeStr=double  OutDataTypeStr=double
  Add1 : Sum  AccumDataTypeStr=double  OutDataTypeStr=double
  Delay{,1..3} (4 alike) : Delay  DelayLength=1  SampleTime=1/44100
  LoR_0 : Constant  Value=0.332670553  OutDataTypeStr=double  SampleTime=1/44100
  LoR_2 : Constant  Value=0.459877502  OutDataTypeStr=double  SampleTime=1/44100
  LoR_4 : Constant  Value=-0.085441274  OutDataTypeStr=double  SampleTime=1/44100
  Multiply : Product  OutDataTypeStr=double
  Multiply1 : Product  OutDataTypeStr=double
  Multiply2 : Product  OutDataTypeStr=double
  Rate Transition : RateTransition  OutPortSampleTime=1/44100
  Rate Transition1 : RateTransition  OutPortSampleTime=1/44100
  Out_LoR_e : Outport  OutDataTypeStr=double  SampleTime=1/44100  VectorParamsAs1DForOutWhenUnconnected=off
  wires:
  Delay/1 -> Rate Transition/1
  Rate Transition1/1 -> Multiply2/2
  Delay2/1 -> Add1/2
  LoR_0/1 -> Multiply/1
  Add/1 -> Out_LoR_e/1
  Delay1/1 -> Rate Transition1/1
  LoR_2/1 -> Multiply1/1
  Multiply1/1 -> Add1/1
  Rate Transition/1 -> Delay1/1, Multiply1/2
  Add1/1 -> Delay3/1
  Multiply/1 -> Add/1
  In_LoR_e/1 -> Delay/1, Multiply/2
  Multiply2/1 -> Delay2/1
  LoR_4/1 -> Multiply2/1
  Delay3/1 -> Add/2

== system db3_7_Level_double/4th_Level_Recon/LoR_Odd ==
  In_LoR_o : Inport  OutDataTypeStr=double  SampleTime=1/44100
  Add : Sum  AccumDataTypeStr=double  OutDataTypeStr=double
  Add1 : Sum  AccumDataTypeStr=double  OutDataTypeStr=double
  Delay{,1..3} (4 alike) : Delay  DelayLength=1  SampleTime=1/44100
  LoR_1 : Constant  Value=0.806891509  OutDataTypeStr=double  SampleTime=1/44100
  LoR_3 : Constant  Value=-0.13501102  OutDataTypeStr=double  SampleTime=1/44100
  LoR_5 : Constant  Value=0.035226292  OutDataTypeStr=double  SampleTime=1/44100
  Multiply : Product  OutDataTypeStr=double
  Multiply1 : Product  OutDataTypeStr=double
  Multiply2 : Product  OutDataTypeStr=double
  Rate Transition : RateTransition  OutPortSampleTime=1/44100
  Rate Transition1 : RateTransition  OutPortSampleTime=1/44100
  Out_LoR_o : Outport  OutDataTypeStr=double  SampleTime=1/44100  VectorParamsAs1DForOutWhenUnconnected=off
  wires:
  Delay/1 -> Rate Transition/1
  Rate Transition1/1 -> Multiply2/2
  Delay2/1 -> Add1/2
  LoR_1/1 -> Multiply/1
  Add/1 -> Out_LoR_o/1
  Delay1/1 -> Rate Transition1/1
  LoR_3/1 -> Multiply1/1
  Multiply1/1 -> Add1/1
  Rate Transition/1 -> Delay1/1, Multiply1/2
  Add1/1 -> Delay3/1
  Multiply/1 -> Add/1
  In_LoR_o/1 -> Delay/1, Multiply/2
  Multiply2/1 -> Delay2/1
  LoR_5/1 -> Multiply2/1
  Delay3/1 -> Add/2

== system db3_7_Level_double/5th_Level_Decomp/HiD_Even ==
  In_HiD_e : Inport  OutDataTypeStr=double  SampleTime=1/44100
  Add : Sum  AccumDataTypeStr=double  OutDataTypeStr=double
  Add1 : Sum  AccumDataTypeStr=double  OutDataTypeStr=double
  Delay{,1..3} (4 alike) : Delay  DelayLength=1  SampleTime=1/44100
  HiD_0 : Constant  Value=-0.332670553  OutDataTypeStr=double  SampleTime=1/44100
  HiD_2 : Constant  Value=-0.459877502  OutDataTypeStr=double  SampleTime=1/44100
  HiD_4 : Constant  Value=0.085441274  OutDataTypeStr=double  SampleTime=1/44100
  Multiply : Product  OutDataTypeStr=double
  Multiply1 : Product  OutDataTypeStr=double
  Multiply2 : Product  OutDataTypeStr=double
  Rate Transition : RateTransition  OutPortSampleTime=1/44100
  Rate Transition1 : RateTransition  OutPortSampleTime=1/44100
  Out_HiD_e : Outport  OutDataTypeStr=double  SampleTime=1/44100  VectorParamsAs1DForOutWhenUnconnected=off
  wires:
  In_HiD_e/1 -> Delay/1, Multiply/2
  Rate Transition/1 -> Delay1/1, Multiply1/2
  HiD_0/1 -> Multiply/1
  HiD_2/1 -> Multiply1/1
  Add/1 -> Out_HiD_e/1
  Rate Transition1/1 -> Multiply2/2
  HiD_4/1 -> Multiply2/1
  Multiply1/1 -> Add1/1
  Multiply2/1 -> Delay2/1
  Delay2/1 -> Add1/2
  Add1/1 -> Delay3/1
  Delay3/1 -> Add/2
  Multiply/1 -> Add/1
  Delay/1 -> Rate Transition/1
  Delay1/1 -> Rate Transition1/1

== system db3_7_Level_double/5th_Level_Decomp/HiD_Odd ==
  In_HiD_o : Inport  OutDataTypeStr=double  SampleTime=1/44100
  Add : Sum  AccumDataTypeStr=double  OutDataTypeStr=double
  Add1 : Sum  AccumDataTypeStr=double  OutDataTypeStr=double
  Delay{,1..3} (4 alike) : Delay  DelayLength=1  SampleTime=1/44100
  HiD_1 : Constant  Value=0.806891509  OutDataTypeStr=double  SampleTime=1/44100
  HiD_3 : Constant  Value=-0.13501102  OutDataTypeStr=double  SampleTime=1/44100
  HiD_5 : Constant  Value=0.035226292  OutDataTypeStr=double  SampleTime=1/44100
  Multiply : Product  OutDataTypeStr=double
  Multiply1 : Product  OutDataTypeStr=double
  Multiply2 : Product  OutDataTypeStr=double
  Rate Transition : RateTransition  OutPortSampleTime=1/44100
  Rate Transition1 : RateTransition  OutPortSampleTime=1/44100
  Out_HiD_o : Outport  OutDataTypeStr=double  SampleTime=1/44100  VectorParamsAs1DForOutWhenUnconnected=off
  wires:
  HiD_5/1 -> Multiply2/1
  HiD_3/1 -> Multiply1/1
  Add/1 -> Out_HiD_o/1
  Delay2/1 -> Add1/2
  Delay3/1 -> Add/2
  Add1/1 -> Delay3/1
  Multiply/1 -> Add/1
  HiD_1/1 -> Multiply/1
  Rate Transition/1 -> Delay1/1, Multiply1/2
  Multiply1/1 -> Add1/1
  Multiply2/1 -> Delay2/1
  Rate Transition1/1 -> Multiply2/2
  In_HiD_o/1 -> Multiply/2, Delay/1
  Delay/1 -> Rate Transition/1
  Delay1/1 -> Rate Transition1/1

== system db3_7_Level_double/5th_Level_Decomp/LoD_Even ==
  In_LoD_e : Inport  OutDataTypeStr=double  SampleTime=1/44100
  Add : Sum  AccumDataTypeStr=double  OutDataTypeStr=double
  Add1 : Sum  AccumDataTypeStr=double  OutDataTypeStr=double
  Delay{,1..3} (4 alike) : Delay  DelayLength=1  SampleTime=1/44100
  LoD_0 : Constant  Value=0.035226292  OutDataTypeStr=double  SampleTime=1/44100
  LoD_2 : Constant  Value=-0.13501102  OutDataTypeStr=double  SampleTime=1/44100
  LoD_4 : Constant  Value=0.806891509  OutDataTypeStr=double  SampleTime=1/44100
  Multiply : Product  OutDataTypeStr=double
  Multiply1 : Product  OutDataTypeStr=double
  Multiply2 : Product  OutDataTypeStr=double
  Rate Transition : RateTransition  OutPortSampleTime=1/44100
  Rate Transition1 : RateTransition  OutPortSampleTime=1/44100
  Out_LoD_e : Outport  OutDataTypeStr=double  SampleTime=1/44100  VectorParamsAs1DForOutWhenUnconnected=off
  wires:
  LoD_4/1 -> Multiply2/1
  LoD_2/1 -> Multiply1/1
  Add/1 -> Out_LoD_e/1
  Delay2/1 -> Add1/2
  Delay3/1 -> Add/2
  Add1/1 -> Delay3/1
  Multiply/1 -> Add/1
  LoD_0/1 -> Multiply/1
  Rate Transition/1 -> Delay1/1, Multiply1/2
  Multiply1/1 -> Add1/1
  Multiply2/1 -> Delay2/1
  Rate Transition1/1 -> Multiply2/2
  In_LoD_e/1 -> Delay/1, Multiply/2
  Delay/1 -> Rate Transition/1
  Delay1/1 -> Rate Transition1/1

== system db3_7_Level_double/5th_Level_Decomp/LoD_Odd ==
  In_LoD_o : Inport  OutDataTypeStr=double  SampleTime=1/44100
  Add : Sum  AccumDataTypeStr=double  OutDataTypeStr=double
  Add1 : Sum  AccumDataTypeStr=double  OutDataTypeStr=double
  Delay{,1..3} (4 alike) : Delay  DelayLength=1  SampleTime=1/44100
  LoD_1 : Constant  Value=-0.085441274  OutDataTypeStr=double  SampleTime=1/44100
  LoD_3 : Constant  Value=0.459877502  OutDataTypeStr=double  SampleTime=1/44100
  LoD_5 : Constant  Value=0.332670553  OutDataTypeStr=double  SampleTime=1/44100
  Multiply : Product  OutDataTypeStr=double
  Multiply1 : Product  OutDataTypeStr=double
  Multiply2 : Product  OutDataTypeStr=double
  Rate Transition : RateTransition  OutPortSampleTime=1/44100
  Rate Transition1 : RateTransition  OutPortSampleTime=1/44100
  Out_LoD_o : Outport  OutDataTypeStr=double  SampleTime=1/44100  VectorParamsAs1DForOutWhenUnconnected=off
  wires:
  LoD_5/1 -> Multiply2/1
  LoD_3/1 -> Multiply1/1
  Add/1 -> Out_LoD_o/1
  Delay2/1 -> Add1/2
  Delay3/1 -> Add/2
  Add1/1 -> Delay3/1
  Multiply/1 -> Add/1
  LoD_1/1 -> Multiply/1
  Rate Transition/1 -> Delay1/1, Multiply1/2
  Multiply1/1 -> Add1/1
  Multiply2/1 -> Delay2/1
  Rate Transition1/1 -> Multiply2/2
  In_LoD_o/1 -> Delay/1, Multiply/2
  Delay/1 -> Rate Transition/1
  Delay1/1 -> Rate Transition1/1

== system db3_7_Level_double/5th_Level_Recon/HiR_Even ==
  In_HiR_e : Inport  OutDataTypeStr=double  SampleTime=1/44100
  Add : Sum  AccumDataTypeStr=double  OutDataTypeStr=double
  Add1 : Sum  AccumDataTypeStr=double  OutDataTypeStr=double
  Delay : Delay  DelayLength=1  SampleTime=1/44100
  Delay1 : Delay  DelayLength=1  SampleTime=1/44100
  Delay2 : Delay  DelayLength=1  SampleTime=0.000022675736
  Delay3 : Delay  DelayLength=1  SampleTime=0.000022675736
  HiR_0 : Constant  Value=0.035226292  OutDataTypeStr=double  SampleTime=1/44100
  HiR_2 : Constant  Value=-0.13501102  OutDataTypeStr=double  SampleTime=1/44100
  HiR_4 : Constant  Value=0.806891509  OutDataTypeStr=double  SampleTime=1/44100
  Multiply : Product  OutDataTypeStr=double
  Multiply1 : Product  OutDataTypeStr=double
  Multiply2 : Product  OutDataTypeStr=double
  Rate Transition : RateTransition  OutPortSampleTime=1/44100
  Rate Transition1 : RateTransition  OutPortSampleTime=1/44100
  Out_HiR_e : Outport  OutDataTypeStr=double  SampleTime=1/44100  VectorParamsAs1DForOutWhenUnconnected=off
  wires:
  Delay3/1 -> Add/2
  In_HiR_e/1 -> Delay/1, Multiply/2
  HiR_4/1 -> Multiply2/1
  Multiply/1 -> Add/1
  Add1/1 -> Delay3/1
  Multiply2/1 -> Delay2/1
  Multiply1/1 -> Add1/1
  Delay2/1 -> Add1/2
  Add/1 -> Out_HiR_e/1
  HiR_0/1 -> Multiply/1
  HiR_2/1 -> Multiply1/1
  Delay1/1 -> Rate Transition1/1
  Rate Transition/1 -> Delay1/1, Multiply1/2
  Rate Transition1/1 -> Multiply2/2
  Delay/1 -> Rate Transition/1
